simulink model "panuzin"  (R2024a)
settings: Solver=VariableStepAuto  StartTime=0.0  StopTime=100  RelTol=1e-3
settings Model: Creator=Lore2  LastModifiedBy=Lore2

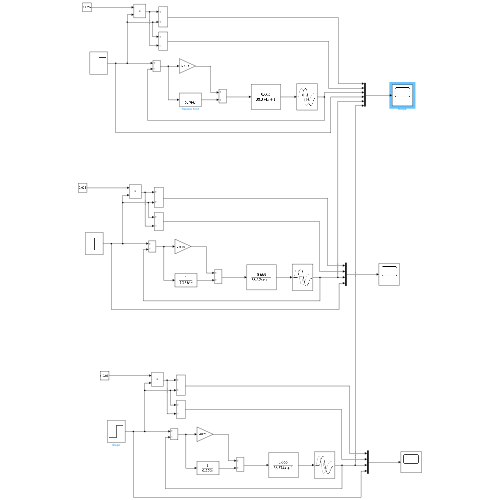
[thumbnail: Simulink's stored preview of the top-level diagram]
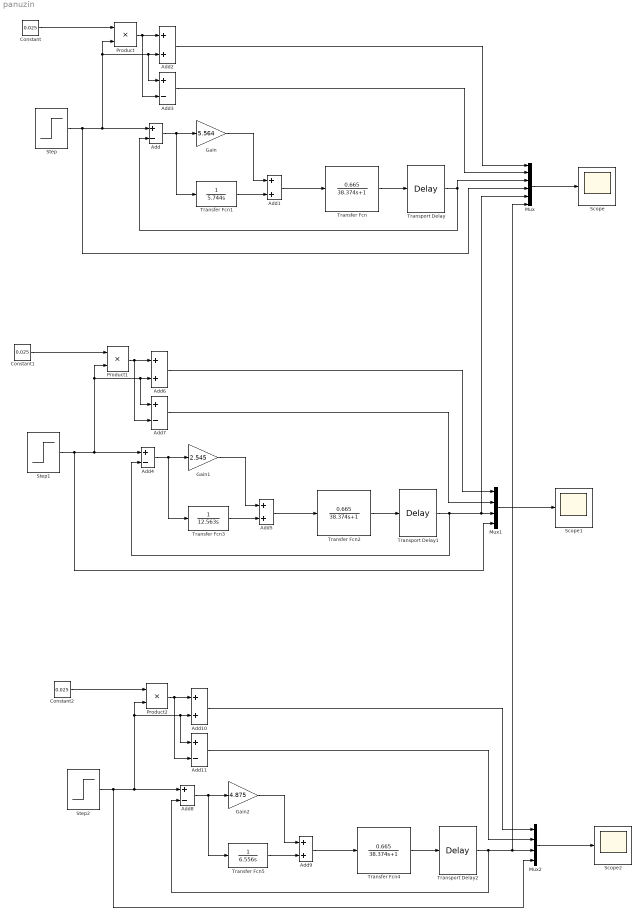
== system panuzin ==
  Add{,3..4,7..8,11} (6 alike) : Sum  Inputs=+-
  Add{1..2,5..6,9..10} (6 alike) : Sum
  Constant : Constant  Value=0.025
  Constant1 : Constant  Value=0.025
  Constant2 : Constant  Value=0.025
  Gain : Gain  Gain=5.564
  Gain1 : Gain  Gain=2.545
  Gain2 : Gain  Gain=4.875
  Mux : Mux  Inputs=6
  Mux1 : Mux
  Mux2 : Mux
  Product : Product
  Product1 : Product
  Product2 : Product
  Scope : Scope
  Scope1 : Scope
  Scope2 : Scope
  Step : Step  After=0.328  SampleTime=0
  Step1 : Step  After=0.328  SampleTime=0
  Step2 : Step  After=0.328  SampleTime=0
  Transfer Fcn : TransferFcn  Numerator=[0.665]  Denominator=[38.374 1]
  Transfer Fcn1 : TransferFcn  Denominator=[5.744 0]
  Transfer Fcn2 : TransferFcn  Numerator=[0.665]  Denominator=[38.374 1]
  Transfer Fcn3 : TransferFcn  Denominator=[12.563 0]
  Transfer Fcn4 : TransferFcn  Numerator=[0.665]  Denominator=[38.374 1]
  Transfer Fcn5 : TransferFcn  Denominator=[6.556 0]
  Transport Delay : TransportDelay  DelayTime=5.631
  Transport Delay1 : TransportDelay  DelayTime=5.631
  Transport Delay2 : TransportDelay  DelayTime=5.631
  wires:
  Step2/1 -> Mux2/4, Add11/1, Add10/2, Product2/2, Add8/1
  Add10/1 -> Mux2/1
  Add8/1 -> Transfer Fcn5/1, Gain2/1
  Add2/1 -> Mux/1
  Add7/1 -> Mux1/2
  Product2/1 -> Add11/2, Add10/1
  Constant2/1 -> Product2/1
  Add5/1 -> Transfer Fcn2/1
  Constant/1 -> Product/1
  Step1/1 -> Mux1/4, Add7/1, Add6/2, Product1/2, Add4/1
  Add1/1 -> Transfer Fcn/1
  Transfer Fcn4/1 -> Transport Delay2/1
  Add11/1 -> Mux2/2
  Gain2/1 -> Add9/1
  Step/1 -> Mux/4, Add3/1, Add2/2, Product/2, Add/1
  Add4/1 -> Transfer Fcn3/1, Gain1/1
  Gain/1 -> Add1/1
  Transport Delay/1 -> Mux/3, Add/2
  Add6/1 -> Mux1/1
  Transfer Fcn2/1 -> Transport Delay1/1
  Mux2/1 -> Scope2/1
  Transfer Fcn/1 -> Transport Delay/1
  Transfer Fcn3/1 -> Add5/2
  Mux1/1 -> Scope1/1
  Transport Delay1/1 -> Mux/5, Mux1/3, Add4/2
  Transport Delay2/1 -> Mux/6, Mux2/3, Add8/2
  Product1/1 -> Add7/2, Add6/1
  Gain1/1 -> Add5/1
  Add9/1 -> Transfer Fcn4/1
  Add3/1 -> Mux/2
  Mux/1 -> Scope/1
  Product/1 -> Add3/2, Add2/1
  Add/1 -> Transfer Fcn1/1, Gain/1
  Transfer Fcn5/1 -> Add9/2
  Transfer Fcn1/1 -> Add1/2
  Constant1/1 -> Product1/1
